simulink model "studyDashboard"  (R2024a)
settings: Solver=VariableStepAuto  StartTime=0.0  StopTime=inf  RelTol=1e-3
libraries: simulink x1
settings Model: Creator=jh2beauty  LastModifiedBy=jh2beauty

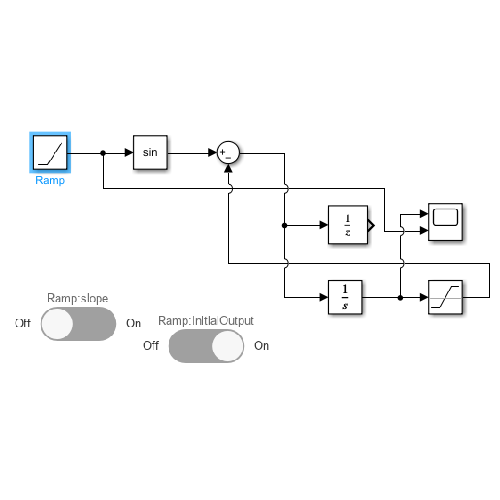
[thumbnail: Simulink's stored preview of the top-level diagram]
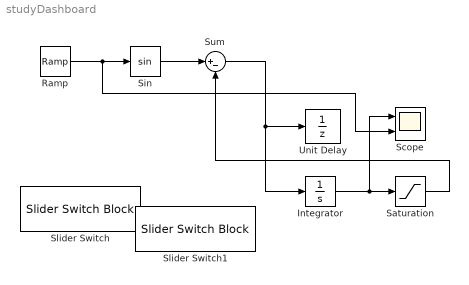
== system studyDashboard ==
  Integrator : Integrator
  Ramp : simulink/Sources/Ramp  slope=-1  start=0  InitialOutput=1
  Saturation : Saturate  UpperLimit=50  LowerLimit=-50
  Scope : Scope  NumInputPorts=2
  Sin : Trigonometry
  Slider Switch : SliderSwitchBlock
      settings: Values={{'Off', 'On'}, [-1 1]}
  Slider Switch1 : SliderSwitchBlock
      settings: Values={{'Off', 'On'}, [-1 1]}
  Sum : Sum  Inputs=|+-
  Unit Delay : UnitDelay  SampleTime=-1  HasFrameUpgradeWarning=on
  wires:
  Sum/1 -> Integrator/1, Unit Delay/1
  Integrator/1 -> Saturation/1, Scope/1
  Saturation/1 -> Sum/2
  Sin/1 -> Sum/1
  Ramp/1 -> Scope/2, Sin/1
